simulink model "oneforall_sim_ob"  (R2017b)
settings: Solver=VariableStepAuto  StartTime=0.0  StopTime=10  RelTol=1e-3
values from neighbouring files (symbols this model uses):
  A = [A11 A12 A13 A14; A21 A22 A23 A24; A31 A32 A33 A34; A41 A42 A43 A44]    [oneforall.m]
  B = [0;0;0;1/jm]    [oneforall.m]
  C = [1 0 0 0]    [oneforall.m]
  L = place(A.',C.',Pob).'    [oneforall.m]
undefined symbols (not defined in the file or in its folder): Kopt
settings Model: Creator=lencs  LastModifiedBy=lencs

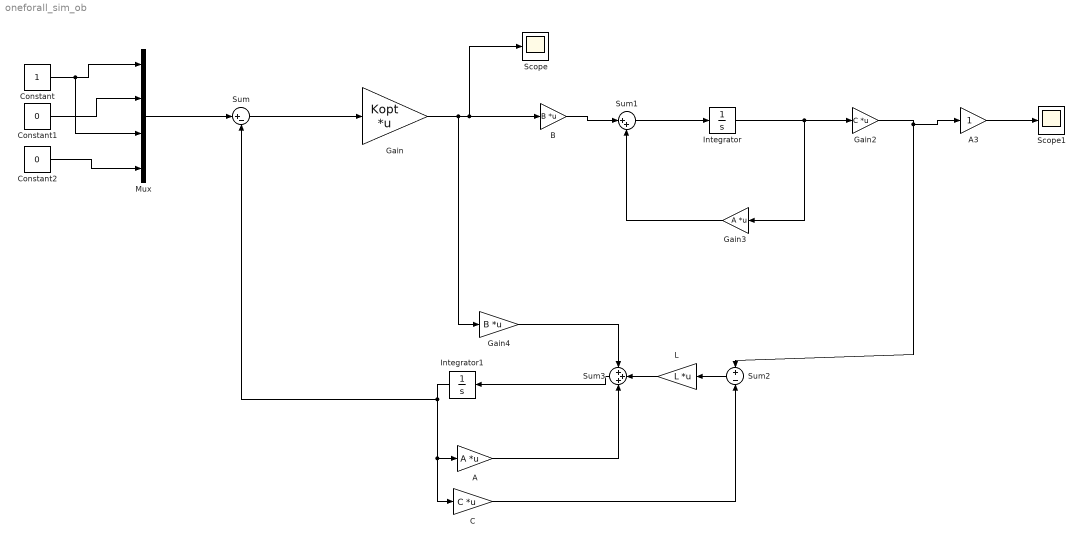
== system oneforall_sim_ob ==
  A : Gain  Gain=A  Multiplication=Matrix(K*u) (u vector)
  "A3 " : Gain
  B : Gain  Gain=B  Multiplication=Matrix(K*u)
  C : Gain  Gain=C  Multiplication=Matrix(K*u)
  Constant : Constant
  Constant1 : Constant  Value=0
  Constant2 : Constant  Value=0
  Gain : Gain  Gain=Kopt  Multiplication=Matrix(K*u)
  Gain2 : Gain  Gain=C  Multiplication=Matrix(K*u)
  Gain3 : Gain  Gain=A  Multiplication=Matrix(K*u) (u vector)
  Gain4 : Gain  Gain=B  Multiplication=Matrix(K*u)
  Integrator : Integrator  InitialCondition=[0.1;0;0;0]
  Integrator1 : Integrator  InitialCondition=[0.05 ;0; 0; 0]
  L : Gain  Gain=L  Multiplication=Matrix(K*u)
  Mux : Mux
  Scope : Scope
  Scope1 : Scope
  Sum : Sum  Inputs=|+-
  Sum1 : Sum  Inputs=|++
  Sum2 : Sum  Inputs=+-
  Sum3 : Sum  Inputs=+++
  wires:
  Constant/1 -> Mux/3, Mux/1
  Constant2/1 -> Mux/4
  Mux/1 -> Sum/1
  Sum/1 -> Gain/1
  Gain/1 -> Gain4/1, Scope/1, B/1
  Sum1/1 -> Integrator/1
  Integrator/1 -> Gain3/1, Gain2/1
  Gain3/1 -> Sum1/2
  B/1 -> Sum1/1
  Constant1/1 -> Mux/2
  A/1 -> Sum3/3
  Sum2/1 -> L/1
  Sum3/1 -> Integrator1/1
  C/1 -> Sum2/2
  L/1 -> Sum3/2
  Integrator1/1 -> Sum/2, C/1, A/1
  Gain4/1 -> Sum3/1
  "A3 "/1 -> Scope1/1
  Gain2/1 -> "A3 "/1, Sum2/1
